simulink model "sudoku_demo"  (R2016b)
settings: Solver=FixedStepDiscrete  StartTime=0.0  StopTime=10.0  RelTol=1e-3
model workspace (MAT data in the model file):
  ContractValidatorBlocksMap = containers.Map
  ContractValidatorBlocksMap.serialization.keys = {'sudoku/contract/validator', 'sudoku_demo/contract/validator'}
  ContractValidatorBlocksMap.serialization.values{1}.block = 'sudoku/contract/validator'
  ContractValidatorBlocksMap.serialization.values{1}.assumePorts = 1
  ContractValidatorBlocksMap.serialization.values{1}.guaranteePorts = 1
  ContractValidatorBlocksMap.serialization.values{1}.modeBlocksPorts = 0
  ContractValidatorBlocksMap.serialization.values{1}.portHandles.Inport = [423.005737305 424.004150391]
  ContractValidatorBlocksMap.serialization.values{1}.portHandles.Outport = 425.013793945
  ContractValidatorBlocksMap.serialization.values{1}.portHandles.Enable = []
  ContractValidatorBlocksMap.serialization.values{1}.portHandles.Trigger = []
  ContractValidatorBlocksMap.serialization.values{1}.portHandles.State = []
  ContractValidatorBlocksMap.serialization.values{1}.portHandles.LConn = []
  ContractValidatorBlocksMap.serialization.values{1}.portHandles.RConn = []
  ContractValidatorBlocksMap.serialization.values{1}.portHandles.Ifaction = []
  ContractValidatorBlocksMap.serialization.values{1}.portHandles.Reset = []
  ContractValidatorBlocksMap.serialization.values{1}.portConnectivity(1).Type = '1'
  ContractValidatorBlocksMap.serialization.values{1}.portConnectivity(1).Position = [385 130]
  ContractValidatorBlocksMap.serialization.values{1}.portConnectivity(1).SrcBlock = 97.0111083984
  ContractValidatorBlocksMap.serialization.values{1}.portConnectivity(1).SrcPort = 0
  ContractValidatorBlocksMap.serialization.values{1}.portConnectivity(1).DstBlock = []
  ContractValidatorBlocksMap.serialization.values{1}.portConnectivity(1).DstPort = []
  ContractValidatorBlocksMap.serialization.values{1}.portConnectivity(2).Type = '2'
  ContractValidatorBlocksMap.serialization.values{1}.portConnectivity(2).Position = [385 270]
  ContractValidatorBlocksMap.serialization.values{1}.portConnectivity(2).SrcBlock = 134.024414062
  ContractValidatorBlocksMap.serialization.values{1}.portConnectivity(2).SrcPort = 0
  ContractValidatorBlocksMap.serialization.values{1}.portConnectivity(2).DstBlock = []
  ContractValidatorBlocksMap.serialization.values{1}.portConnectivity(2).DstPort = []
  ContractValidatorBlocksMap.serialization.values{1}.portConnectivity(3).Type = '1'
  ContractValidatorBlocksMap.serialization.values{1}.portConnectivity(3).Position = [500 200]
  ContractValidatorBlocksMap.serialization.values{1}.portConnectivity(3).SrcBlock = []
  ContractValidatorBlocksMap.serialization.values{1}.portConnectivity(3).SrcPort = []
  ContractValidatorBlocksMap.serialization.values{1}.portConnectivity(3).DstBlock = 409.010986328
  ContractValidatorBlocksMap.serialization.values{1}.portConnectivity(3).DstPort = 0
  ContractValidatorBlocksMap.serialization.values{2}.block = 'sudoku_demo/contract/validator'
  ContractValidatorBlocksMap.serialization.values{2}.assumePorts = 1
  ContractValidatorBlocksMap.serialization.values{2}.guaranteePorts = 1
  ContractValidatorBlocksMap.serialization.values{2}.modeBlocksPorts = 0
  ContractValidatorBlocksMap.serialization.values{2}.portHandles.Inport = [2813.00085449 2814.00085449]
  ContractValidatorBlocksMap.serialization.values{2}.portHandles.Outport = 2815.00085449
  ContractValidatorBlocksMap.serialization.values{2}.portHandles.Enable = []
  ContractValidatorBlocksMap.serialization.values{2}.portHandles.Trigger = []
  ContractValidatorBlocksMap.serialization.values{2}.portHandles.State = []
  ContractValidatorBlocksMap.serialization.values{2}.portHandles.LConn = []
  ContractValidatorBlocksMap.serialization.values{2}.portHandles.RConn = []
  ContractValidatorBlocksMap.serialization.values{2}.portHandles.Ifaction = []
  ContractValidatorBlocksMap.serialization.values{2}.portHandles.Reset = []
  ContractValidatorBlocksMap.serialization.values{2}.portConnectivity(1).Type = '1'
  ContractValidatorBlocksMap.serialization.values{2}.portConnectivity(1).Position = [355 130]
  ContractValidatorBlocksMap.serialization.values{2}.portConnectivity(1).SrcBlock = 14.0013427734
  ContractValidatorBlocksMap.serialization.values{2}.portConnectivity(1).SrcPort = 0
  ContractValidatorBlocksMap.serialization.values{2}.portConnectivity(1).DstBlock = []
  ContractValidatorBlocksMap.serialization.values{2}.portConnectivity(1).DstPort = []
  ContractValidatorBlocksMap.serialization.values{2}.portConnectivity(2).Type = '2'
  ContractValidatorBlocksMap.serialization.values{2}.portConnectivity(2).Position = [355 270]
  ContractValidatorBlocksMap.serialization.values{2}.portConnectivity(2).SrcBlock = 30.0017089844
  ContractValidatorBlocksMap.serialization.values{2}.portConnectivity(2).SrcPort = 0
  ContractValidatorBlocksMap.serialization.values{2}.portConnectivity(2).DstBlock = []
  ContractValidatorBlocksMap.serialization.values{2}.portConnectivity(2).DstPort = []
  ContractValidatorBlocksMap.serialization.values{2}.portConnectivity(3).Type = '1'
  ContractValidatorBlocksMap.serialization.values{2}.portConnectivity(3).Position = [435 200]
  ContractValidatorBlocksMap.serialization.values{2}.portConnectivity(3).SrcBlock = []
  ContractValidatorBlocksMap.serialization.values{2}.portConnectivity(3).SrcPort = []
  ContractValidatorBlocksMap.serialization.values{2}.portConnectivity(3).DstBlock = 2800.00109863
  ContractValidatorBlocksMap.serialization.values{2}.portConnectivity(3).DstPort = 0
  ContractValidatorBlocksMap.serialization.uniformity = 0
  ContractValidatorBlocksMap.serialization.keyType = 'char'
  ContractValidatorBlocksMap.serialization.valueType = 'any'
undefined symbols (not defined in the file): contractAfterSimulation, ContractAssumeBlock, contractBeforeSimulation, ContractBlock, ContractGuaranteeBlock, ContractValidatorBlock, saveValidatorParameters
libraries: simulink x30
settings Model: Creator=hbourbou  LastModifiedBy=hbourbou

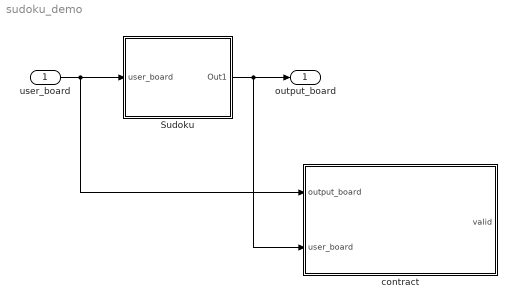
== system sudoku_demo ==
  user_board : Inport  OutDataTypeStr=uint8  PortDimensions=[9,9]
  Sudoku : Subsystem
  contract : Subsystem  mask(ContractBlock){ContractBlockType=ContractBlock}
      mask init:
      | set_param(gcb, 'LinkStatus', 'none');
      settings: CopyFcn=set_param(gcb, 'LinkStatus', 'none');
      mask DialogControl DescTextVar Prompt: Contract block
      mask Display:
      | text(0.5, 0.5, '{\bf\fontsize{20}Contract}', 'hor', 'center', 'texmode','on');
      | blocks = find_system(gcb, 'LookUnderMasks','all', 'SearchDepth',1,'BlockType','Inport');
      | for i = 1 : length(blocks)
      |     blockName = get_param(blocks(i), 'Name');
      |     [path, blockName] = fileparts(char(blockName));
      |     port_label('input', i, blockName);
      | end
      | 
      | blocks = find_system(gcb, 'LookUnderMasks','all', 'SearchDepth',1,'BlockType','Outport');
      | for i = 1 : length(blocks)
      |     blockName = get_param(blocks(i), 'Name');
      |     [path, blockName] = fileparts(char(blockName));
      |     port_label('output', i, blockName);
      | end
  output_board : Outport
  wires:
  Sudoku/1(Out1) -> contract/2(user_board), output_board/1
  user_board/1 -> contract/1(output_board), Sudoku/1(user_board)

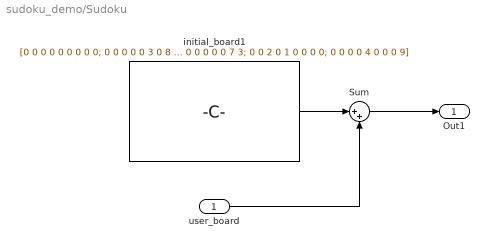
== system sudoku_demo/Sudoku ==
  user_board : Inport
  Sum : Sum  Inputs=|++
  initial_board1 : Constant  Value=[0 0 0 0 0 0 0 0 0; 0 0 0 0 0 3 0 8 5; 0 0 1 0 2 0 0 0 0; 0 0 0 5 0 7 0 0 0; 0 0 4 0 0 0 1 0 0; 0 9 0 0 0 0 0 0 0; 5 0 0 0 0 0 0 7 3; 0 0 2 0 1 0 0 0 0; 0 0 0 0 4 0 0 0 9]  OutDataTypeStr=uint8
  Out1 : Outport
  wires:
  user_board/1 -> Sum/2
  initial_board1/1 -> Sum/1
  Sum/1 -> Out1/1

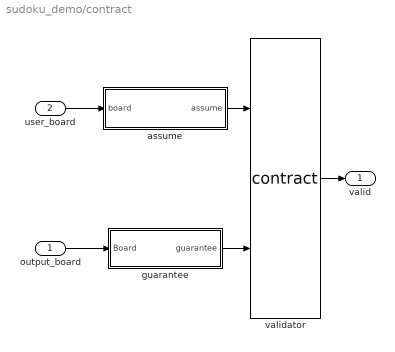
== system sudoku_demo/contract ==
  output_board : Inport
  user_board : Inport  Port=2
  assume : Subsystem  mask(ContractAssumeBlock){ContractBlockType=ContractAssumeBlock}
      mask init:
      | set_param(gcb, 'LinkStatus', 'none');
      mask DialogControl DescTextVar Prompt: Assume block
  guarantee : Subsystem  mask(ContractGuaranteeBlock){ContractBlockType=ContractGuaranteeBlock}
      mask init:
      | set_param(gcb, 'LinkStatus', 'none');
      mask DialogControl DescTextVar Prompt: Guarantee block
  validator : M-S-Function  LoadFcn=saveValidatorParameters(gcb);  InitFcn=contractBeforeSimulation();  StopFcn=contractAfterSimulation();  FunctionName=contract  mask(ContractValidatorBlock){assumePorts=1, guaranteePorts=1, modePorts=0, ContractBlockType=ContractValidatorBlock, createInportsCheckbox=off}
      mask prompts: assumePorts "Assume ports     :"; guaranteePorts "Guarantee ports :"; modePorts "Mode ports        :"; createInportsCheckbox "Create inports and connect them automatically"
      mask init:
      | set_param(gcb,'LinkStatus','none');
      | contract_callback('inputs_callback',gcb);
      mask DialogControl DescTextVar Prompt: The validator block implements the following logic: <br> <br> <b>Sofar</b>(assume<sub>1</sub> <b>&#8743;</b> assume<sub>2</sub> <b>&#8743;</b> ... assume<sub>k</sub>) <b>&rarr;</b> (guarantee<sub>1</sub> <b>&#8743;</b> guarantee<sub>2</sub> <b>&#8743;</b> ... guarantee<sub>m</sub> <b>&#8743;</b>  mode<sub>1</sub> <b>&#8743;</b> mode<sub>2</sub> <b>&#8743;</b> ... <b>&#8743;</b> mode<sub>n</sub> )<br> where mode<sub>i</sub> = require<sub>i</sub> <b>&rarr;</b> ensure<sub>i</sub>
      mask Display:
      | color('black');
      | port_label('input',1,'assume');
      | port_label('input',2,'guarantee');
      | port_label('output',1,'valid');
  valid : Outport
  wires:
  output_board/1 -> guarantee/1(Board)
  validator/1 -> valid/1
  guarantee/1(guarantee) -> validator/2
  assume/1(assume) -> validator/1
  user_board/1 -> assume/1(board)

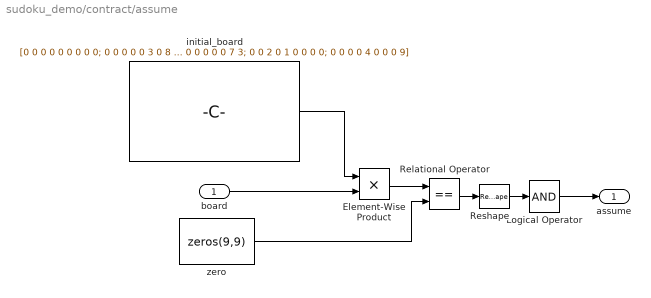
== system sudoku_demo/contract/assume ==
  board : Inport
  Element-Wise Product : Product
  Logical Operator : Logic  Inputs=1  AllPortsSameDT=off  OutDataTypeStr=boolean
  Relational Operator : RelationalOperator  Operator===  OutDataTypeStr=boolean  RndMeth=Simplest
  Reshape : Reshape
  initial_board : Constant  Value=[0 0 0 0 0 0 0 0 0; 0 0 0 0 0 3 0 8 5; 0 0 1 0 2 0 0 0 0; 0 0 0 5 0 7 0 0 0; 0 0 4 0 0 0 1 0 0; 0 9 0 0 0 0 0 0 0; 5 0 0 0 0 0 0 7 3; 0 0 2 0 1 0 0 0 0; 0 0 0 0 4 0 0 0 9]  OutDataTypeStr=uint8
  zero : Constant  Value=zeros(9,9)  OutDataTypeStr=uint8
  assume : Outport  OutDataTypeStr=boolean
  wires:
  initial_board/1 -> Element-Wise Product/1
  board/1 -> Element-Wise Product/2
  Element-Wise Product/1 -> Relational Operator/1
  zero/1 -> Relational Operator/2
  Relational Operator/1 -> Reshape/1
  Logical Operator/1 -> assume/1
  Reshape/1 -> Logical Operator/1

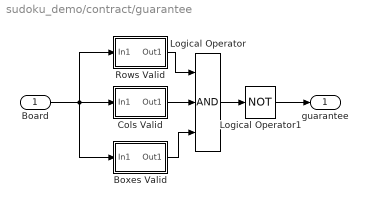
== system sudoku_demo/contract/guarantee ==
  Board : Inport  PortDimensions=[9 9]
  Boxes Valid : Subsystem
  Cols Valid : Subsystem
  Logical Operator : Logic  Inputs=3  AllPortsSameDT=off  OutDataTypeStr=boolean
  Logical Operator1 : Logic  Operator=NOT  AllPortsSameDT=off  OutDataTypeStr=boolean
  Rows Valid : Subsystem
  guarantee : Outport  OutDataTypeStr=boolean
  wires:
  Board/1 -> Boxes Valid/1(In1), Rows Valid/1(In1), Cols Valid/1(In1)
  Rows Valid/1(Out1) -> Logical Operator/1
  Cols Valid/1(Out1) -> Logical Operator/2
  Boxes Valid/1(Out1) -> Logical Operator/3
  Logical Operator/1 -> Logical Operator1/1
  Logical Operator1/1 -> guarantee/1

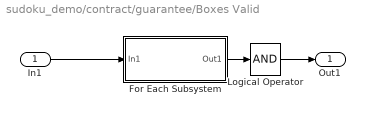
== system sudoku_demo/contract/guarantee/Boxes Valid ==
  In1 : Inport
  For Each Subsystem : Subsystem  TreatAsAtomicUnit=on
  Logical Operator : Logic  Inputs=1  AllPortsSameDT=off  OutDataTypeStr=boolean
  Out1 : Outport
  wires:
  In1/1 -> For Each Subsystem/1(In1)
  For Each Subsystem/1(Out1) -> Logical Operator/1
  Logical Operator/1 -> Out1/1

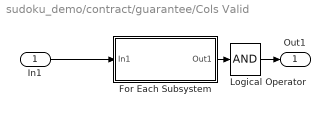
== system sudoku_demo/contract/guarantee/Cols Valid ==
  In1 : Inport
  For Each Subsystem : Subsystem  TreatAsAtomicUnit=on
  Logical Operator : Logic  Inputs=1  AllPortsSameDT=off  OutDataTypeStr=boolean
  Out1 : Outport
  wires:
  In1/1 -> For Each Subsystem/1(In1)
  For Each Subsystem/1(Out1) -> Logical Operator/1
  Logical Operator/1 -> Out1/1

== system sudoku_demo/contract/guarantee/Rows Valid ==
  In1 : Inport
  For Each Subsystem : Subsystem  TreatAsAtomicUnit=on
  Logical Operator : Logic  Inputs=1  AllPortsSameDT=off  OutDataTypeStr=boolean
  Out1 : Outport
  wires:
  In1/1 -> For Each Subsystem/1(In1)
  For Each Subsystem/1(Out1) -> Logical Operator/1
  Logical Operator/1 -> Out1/1

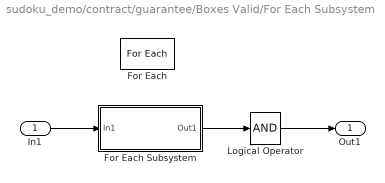
== system sudoku_demo/contract/guarantee/Boxes Valid/For Each Subsystem ==
  In1 : Inport  Partition=on  PartitionDimension=1  PartitionWidth=3
  For Each : ForEach  DisableCoverage=on
  For Each Subsystem : Subsystem  TreatAsAtomicUnit=on
  Logical Operator : Logic  Inputs=1  AllPortsSameDT=off  OutDataTypeStr=boolean
  Out1 : Outport  ConcatenationDimension=1
  wires:
  In1/1 -> For Each Subsystem/1(In1)
  Logical Operator/1 -> Out1/1
  For Each Subsystem/1(Out1) -> Logical Operator/1

== system sudoku_demo/contract/guarantee/Cols Valid/For Each Subsystem ==
  In1 : Inport  Partition=on  PartitionDimension=2  PartitionWidth=1
  For Each : ForEach  DisableCoverage=on
  Vector is valid : Subsystem
  Out1 : Outport  ConcatenationDimension=1
  wires:
  In1/1 -> Vector is valid/1(In1)
  Vector is valid/1(Out1) -> Out1/1

== system sudoku_demo/contract/guarantee/Rows Valid/For Each Subsystem ==
  In1 : Inport  Partition=on  PartitionDimension=1  PartitionWidth=1
  For Each : ForEach  DisableCoverage=on
  Vector is valid : Subsystem
  Out1 : Outport  ConcatenationDimension=1
  wires:
  In1/1 -> Vector is valid/1(In1)
  Vector is valid/1(Out1) -> Out1/1

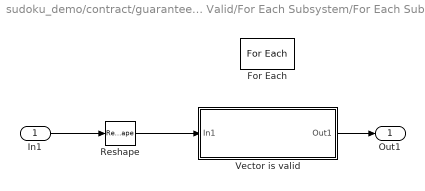
== system sudoku_demo/contract/guarantee/Boxes Valid/For Each Subsystem/For Each Subsystem ==
  In1 : Inport  Partition=on  PartitionDimension=2  PartitionWidth=3
  For Each : ForEach  DisableCoverage=on
  Reshape : Reshape
  Vector is valid : Subsystem
  Out1 : Outport  ConcatenationDimension=1
  wires:
  In1/1 -> Reshape/1
  Vector is valid/1(Out1) -> Out1/1
  Reshape/1 -> Vector is valid/1(In1)

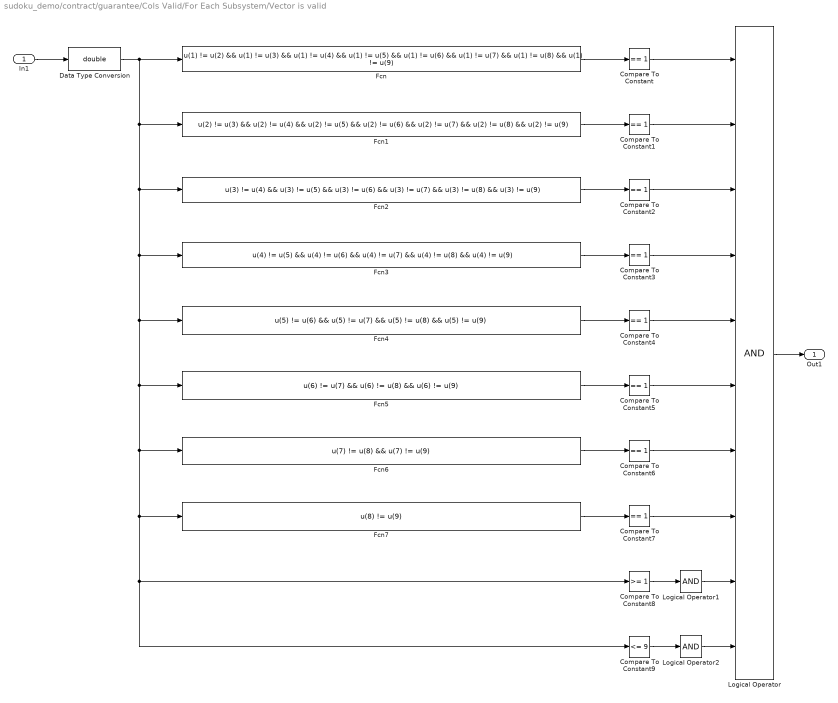
== system sudoku_demo/contract/guarantee/Cols Valid/For Each Subsystem/Vector is valid ==
  In1 : Inport
  Compare To Constant{,1..7} (8 alike) : simulink/Logic and Bit Operations/Compare To Constant  relop===  const=1  OutDataTypeStr=boolean
  Compare To Constant8 : simulink/Logic and Bit Operations/Compare To Constant  relop=>=  const=1  OutDataTypeStr=boolean
  Compare To Constant9 : simulink/Logic and Bit Operations/Compare To Constant  relop=<=  const=9  OutDataTypeStr=boolean
  Data Type Conversion : DataTypeConversion  OutDataTypeStr=double
  Fcn : Fcn  Expr=u(1) != u(2) && u(1) != u(3) && u(1) != u(4) && u(1) != u(5) && u(1) != u(6) && u(1) != u(7) && u(1) != u(8) && u(1) != u(9)
  Fcn1 : Fcn  Expr=u(2) != u(3) && u(2) != u(4) && u(2) != u(5) && u(2) != u(6) && u(2) != u(7) && u(2) != u(8) && u(2) != u(9)
  Fcn2 : Fcn  Expr=u(3) != u(4) && u(3) != u(5) && u(3) != u(6) && u(3) != u(7) && u(3) != u(8) && u(3) != u(9)
  Fcn3 : Fcn  Expr=u(4) != u(5) && u(4) != u(6) && u(4) != u(7) && u(4) != u(8) && u(4) != u(9)
  Fcn4 : Fcn  Expr=u(5) != u(6) && u(5) != u(7) && u(5) != u(8) && u(5) != u(9)
  Fcn5 : Fcn  Expr=u(6) != u(7) && u(6) != u(8) && u(6) != u(9)
  Fcn6 : Fcn  Expr=u(7) != u(8) && u(7) != u(9)
  Fcn7 : Fcn  Expr=u(8) != u(9)
  Logical Operator : Logic  Inputs=10  AllPortsSameDT=off  OutDataTypeStr=boolean
  Logical Operator1 : Logic  Inputs=1  AllPortsSameDT=off  OutDataTypeStr=boolean
  Logical Operator2 : Logic  Inputs=1  AllPortsSameDT=off  OutDataTypeStr=boolean
  Out1 : Outport
  wires:
  Fcn6/1 -> Compare To Constant6/1
  Compare To Constant4/1 -> Logical Operator/5
  Fcn3/1 -> Compare To Constant3/1
  Compare To Constant2/1 -> Logical Operator/3
  Fcn4/1 -> Compare To Constant4/1
  Compare To Constant3/1 -> Logical Operator/4
  Logical Operator/1 -> Out1/1
  Compare To Constant/1 -> Logical Operator/1
  Compare To Constant6/1 -> Logical Operator/7
  Fcn1/1 -> Compare To Constant1/1
  Fcn/1 -> Compare To Constant/1
  Fcn7/1 -> Compare To Constant7/1
  Fcn2/1 -> Compare To Constant2/1
  In1/1 -> Data Type Conversion/1
  Fcn5/1 -> Compare To Constant5/1
  Compare To Constant5/1 -> Logical Operator/6
  Compare To Constant7/1 -> Logical Operator/8
  Compare To Constant1/1 -> Logical Operator/2
  Compare To Constant8/1 -> Logical Operator1/1
  Logical Operator1/1 -> Logical Operator/9
  Logical Operator2/1 -> Logical Operator/10
  Compare To Constant9/1 -> Logical Operator2/1
  Data Type Conversion/1 -> Fcn/1, Fcn1/1, Fcn2/1, Fcn4/1, Fcn5/1, Compare To Constant9/1, Compare To Constant8/1, Fcn7/1, Fcn6/1, Fcn3/1

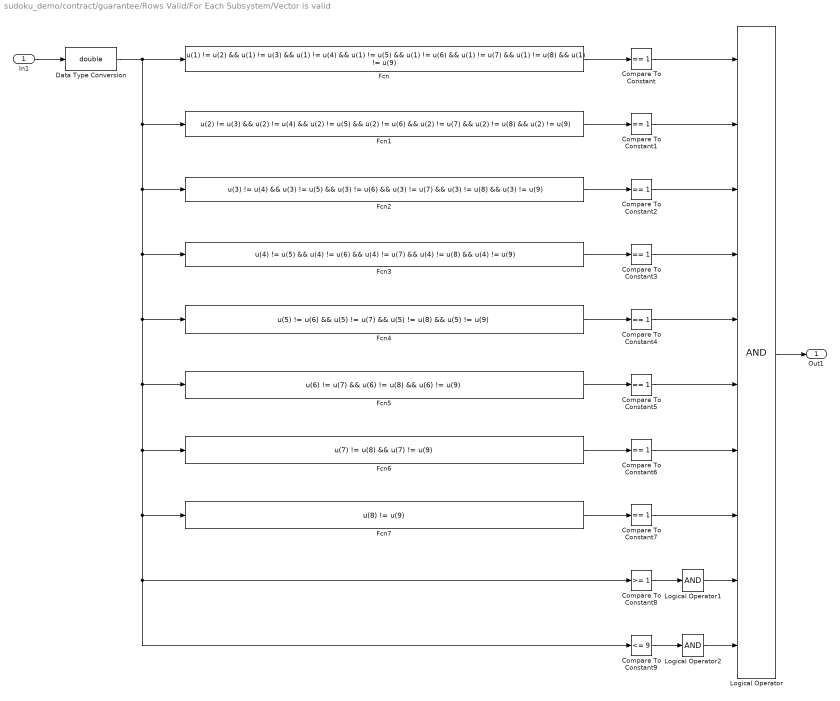
== system sudoku_demo/contract/guarantee/Rows Valid/For Each Subsystem/Vector is valid ==
  In1 : Inport
  Compare To Constant{,1..7} (8 alike) : simulink/Logic and Bit Operations/Compare To Constant  relop===  const=1  OutDataTypeStr=boolean
  Compare To Constant8 : simulink/Logic and Bit Operations/Compare To Constant  relop=>=  const=1  OutDataTypeStr=boolean
  Compare To Constant9 : simulink/Logic and Bit Operations/Compare To Constant  relop=<=  const=9  OutDataTypeStr=boolean
  Data Type Conversion : DataTypeConversion  OutDataTypeStr=double
  Fcn : Fcn  Expr=u(1) != u(2) && u(1) != u(3) && u(1) != u(4) && u(1) != u(5) && u(1) != u(6) && u(1) != u(7) && u(1) != u(8) && u(1) != u(9)
  Fcn1 : Fcn  Expr=u(2) != u(3) && u(2) != u(4) && u(2) != u(5) && u(2) != u(6) && u(2) != u(7) && u(2) != u(8) && u(2) != u(9)
  Fcn2 : Fcn  Expr=u(3) != u(4) && u(3) != u(5) && u(3) != u(6) && u(3) != u(7) && u(3) != u(8) && u(3) != u(9)
  Fcn3 : Fcn  Expr=u(4) != u(5) && u(4) != u(6) && u(4) != u(7) && u(4) != u(8) && u(4) != u(9)
  Fcn4 : Fcn  Expr=u(5) != u(6) && u(5) != u(7) && u(5) != u(8) && u(5) != u(9)
  Fcn5 : Fcn  Expr=u(6) != u(7) && u(6) != u(8) && u(6) != u(9)
  Fcn6 : Fcn  Expr=u(7) != u(8) && u(7) != u(9)
  Fcn7 : Fcn  Expr=u(8) != u(9)
  Logical Operator : Logic  Inputs=10  AllPortsSameDT=off  OutDataTypeStr=boolean
  Logical Operator1 : Logic  Inputs=1  AllPortsSameDT=off  OutDataTypeStr=boolean
  Logical Operator2 : Logic  Inputs=1  AllPortsSameDT=off  OutDataTypeStr=boolean
  Out1 : Outport
  wires:
  Fcn6/1 -> Compare To Constant6/1
  Compare To Constant4/1 -> Logical Operator/5
  Fcn3/1 -> Compare To Constant3/1
  Compare To Constant2/1 -> Logical Operator/3
  Fcn4/1 -> Compare To Constant4/1
  Compare To Constant3/1 -> Logical Operator/4
  Logical Operator/1 -> Out1/1
  Compare To Constant/1 -> Logical Operator/1
  Compare To Constant6/1 -> Logical Operator/7
  Fcn1/1 -> Compare To Constant1/1
  Fcn/1 -> Compare To Constant/1
  Fcn7/1 -> Compare To Constant7/1
  Fcn2/1 -> Compare To Constant2/1
  In1/1 -> Data Type Conversion/1
  Fcn5/1 -> Compare To Constant5/1
  Compare To Constant5/1 -> Logical Operator/6
  Compare To Constant7/1 -> Logical Operator/8
  Compare To Constant1/1 -> Logical Operator/2
  Compare To Constant8/1 -> Logical Operator1/1
  Logical Operator1/1 -> Logical Operator/9
  Logical Operator2/1 -> Logical Operator/10
  Compare To Constant9/1 -> Logical Operator2/1
  Data Type Conversion/1 -> Fcn/1, Fcn1/1, Fcn2/1, Fcn4/1, Fcn5/1, Compare To Constant9/1, Compare To Constant8/1, Fcn7/1, Fcn6/1, Fcn3/1

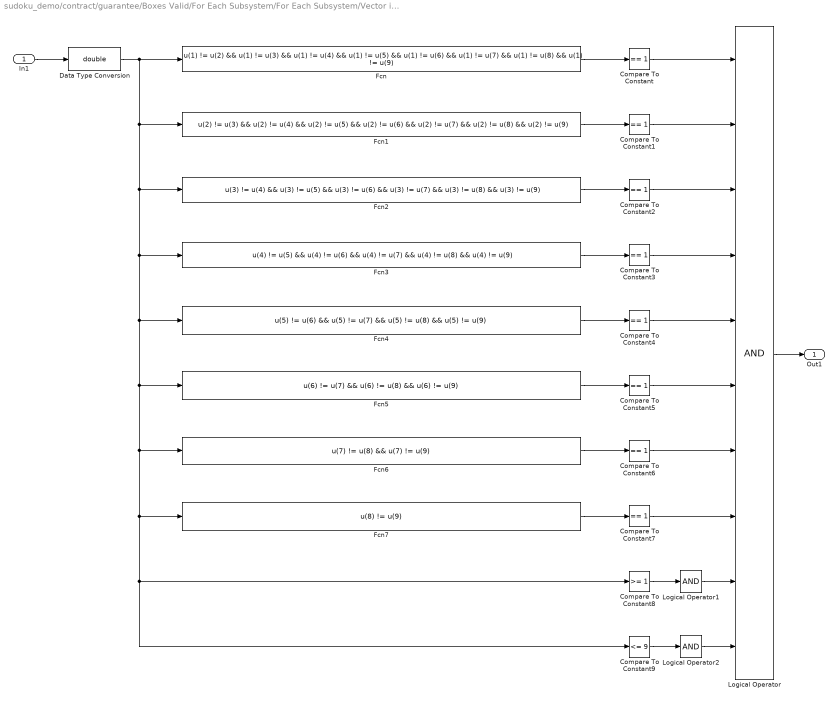
== system sudoku_demo/contract/guarantee/Boxes Valid/For Each Subsystem/For Each Subsystem/Vector is valid ==
  In1 : Inport
  Compare To Constant{,1..7} (8 alike) : simulink/Logic and Bit Operations/Compare To Constant  relop===  const=1  OutDataTypeStr=boolean
  Compare To Constant8 : simulink/Logic and Bit Operations/Compare To Constant  relop=>=  const=1  OutDataTypeStr=boolean
  Compare To Constant9 : simulink/Logic and Bit Operations/Compare To Constant  relop=<=  const=9  OutDataTypeStr=boolean
  Data Type Conversion : DataTypeConversion  OutDataTypeStr=double
  Fcn : Fcn  Expr=u(1) != u(2) && u(1) != u(3) && u(1) != u(4) && u(1) != u(5) && u(1) != u(6) && u(1) != u(7) && u(1) != u(8) && u(1) != u(9)
  Fcn1 : Fcn  Expr=u(2) != u(3) && u(2) != u(4) && u(2) != u(5) && u(2) != u(6) && u(2) != u(7) && u(2) != u(8) && u(2) != u(9)
  Fcn2 : Fcn  Expr=u(3) != u(4) && u(3) != u(5) && u(3) != u(6) && u(3) != u(7) && u(3) != u(8) && u(3) != u(9)
  Fcn3 : Fcn  Expr=u(4) != u(5) && u(4) != u(6) && u(4) != u(7) && u(4) != u(8) && u(4) != u(9)
  Fcn4 : Fcn  Expr=u(5) != u(6) && u(5) != u(7) && u(5) != u(8) && u(5) != u(9)
  Fcn5 : Fcn  Expr=u(6) != u(7) && u(6) != u(8) && u(6) != u(9)
  Fcn6 : Fcn  Expr=u(7) != u(8) && u(7) != u(9)
  Fcn7 : Fcn  Expr=u(8) != u(9)
  Logical Operator : Logic  Inputs=10  AllPortsSameDT=off  OutDataTypeStr=boolean
  Logical Operator1 : Logic  Inputs=1  AllPortsSameDT=off  OutDataTypeStr=boolean
  Logical Operator2 : Logic  Inputs=1  AllPortsSameDT=off  OutDataTypeStr=boolean
  Out1 : Outport
  wires:
  Fcn6/1 -> Compare To Constant6/1
  Compare To Constant4/1 -> Logical Operator/5
  Fcn3/1 -> Compare To Constant3/1
  Compare To Constant2/1 -> Logical Operator/3
  Fcn4/1 -> Compare To Constant4/1
  Compare To Constant3/1 -> Logical Operator/4
  Logical Operator/1 -> Out1/1
  Compare To Constant/1 -> Logical Operator/1
  Compare To Constant6/1 -> Logical Operator/7
  Fcn1/1 -> Compare To Constant1/1
  Fcn/1 -> Compare To Constant/1
  Fcn7/1 -> Compare To Constant7/1
  Fcn2/1 -> Compare To Constant2/1
  In1/1 -> Data Type Conversion/1
  Fcn5/1 -> Compare To Constant5/1
  Compare To Constant5/1 -> Logical Operator/6
  Compare To Constant7/1 -> Logical Operator/8
  Compare To Constant1/1 -> Logical Operator/2
  Compare To Constant8/1 -> Logical Operator1/1
  Logical Operator1/1 -> Logical Operator/9
  Logical Operator2/1 -> Logical Operator/10
  Compare To Constant9/1 -> Logical Operator2/1
  Data Type Conversion/1 -> Fcn/1, Fcn1/1, Fcn2/1, Fcn4/1, Fcn5/1, Compare To Constant9/1, Compare To Constant8/1, Fcn7/1, Fcn6/1, Fcn3/1
